simulink model "VCMGCM1962020b_v2"  (R2020b)
settings: Solver=FixedStepDiscrete  StartTime=0.0  StopTime=10.0  FixedStep=0.005  RelTol=1e-3  EnableMultiTasking=on
PreLoadFcn:
  | try, model_open; catch, disp('Error occurred while executing model pre-load callback: model_open.m'); disp('Please assure that the MATLAB working directory is set to the model directory before opening.'); end
InitFcn:
  | try, model_open; catch, end
undefined symbols (not defined in the file): Bridge, GCM, H, raptor_get_param_eval, raptor_get_safe_string, raptor_xcp_function
libraries: Blocks_lib x1165, Raptor_lib x665, simulink x62, VCM_lib x5
(part 15 of 23)

== system VCMGCM1962020b_v2/Fgnd/Actuators/CAN/CCS Interface/CCSEV_DC_ChargeInfo1/MsgTx ==
  Data : Inport
  Cmd : Inport  Port=2
  Enable : EnablePort
  Bus Selector : BusSelector  OutputSignals=VirtualSensors.Batt.BattSOC [%]
  Bus Selector1 : BusSelector  OutputSignals=EVTargetVoltage [V],EVTargetCurrent [A]
  CANTxField : Blocks_lib/CANTxField  custom=on  custom_nam=[nam '---']  custom_units='---'
  CANTxField1 : Blocks_lib/CANTxField  custom=on  custom_nam=[nam '---']  custom_units='---'
  CANTxField2 : Blocks_lib/CANTxField  custom=on  custom_nam=[nam '---']  custom_units='---'
  Header : Blocks_lib/Header  width=Landscape  addtext=''
  NO_ERROR : Constant  Value=uint8(0)
  RemainingTime : Subsystem
      settings: OpenFcn=open_system(gcb,'force')
  raptor_can_txmsg : Raptor_lib/CAN/raptor_can_txmsg  canDefinition=struct('dbcFile', 'm2iev-api.dbc','message', 'EV_DC_ChargeInfo1','comment', 'EV_DC_ChargeInfo1','signals', {{'EVErrorCode','EVRESSSOC','EVTargetVoltage','EVTargetCurrent','RemainingTimeToFullSoC','RemainingTimeToBulkSoC'}},'enabled', [ 1 1 1 1 1 1;],'canBus', 'bus','messageID', [ 256;],'idMask', [ 536870911;],'payloadMask', [],'payloadValue', [],'period', [ 50;],'mailbox', '''''','queueSize', [ 1;],'label', [ 1;],'ver', [ 2;],'showID', [ 0;],'showRaw', [ 0;],'fill', [ 0;],'editID', [ 0;],'signalOrder', [ 3;])  canBus=bus  queueSize=1  payloadMask=[]  payloadValue=[]  period=50  showID=0  label=1  idMask=hex2dec('1FFFFFFF')  fill=0  id=256  showRaw=0  signalOrder=3  signalInfo={{struct('Name', 'EVErrorCode','Startbit', [ 0;],'SignalSize', [ 4;],'ByteOrder', 'LittleEndian','ValueType', 'UNSIGNED','Class', 'uint8','Signed', [ 0;],'Factor', [ 1;],'Offset', [ 0;],'Min', [ 0;],'Max', [ 11;],'Units', 'Enum','Comment', 'Internal EV error code reported to EVSE','StartBit', [ 4;]),struct('Name', 'EVRESSSOC','Startbit', [ 0;],'SignalSize', [ 8;],'ByteOrder', 'LittleEndian','ValueType', 'UNSIGNED','Class', 'uint8','Signed', [ 0;],'Factor', [ 0.5;],'Offset', [ 0;],'Min', [ 0;],'Max', [ 127.5;],'Units', '%','Comment', 'Current state of charge','StartBit', [ 8;]),struct('Name', 'EVTargetVoltage','Startbit', [ 0;],'SignalSize', [ 16;],'ByteOrder', 'LittleEndian','ValueType', 'UNSIGNED','Class', 'uint16','Signed', [ 0;],'Factor', [ 0.05;],'Offset', [ 0;],'Min', [ 0;],'Max', [ 3276.75;],'Units', 'V','Comment', 'Voltage to be supplied by EVSE','StartBit', [ 16;]),struct('Name', 'EVTargetCurrent','Startbit', [ 0;],'SignalSize', [ 16;],'ByteOrder', 'LittleEndian','ValueType', 'SIGNED','Class', 'int16','Signed', [ 1;],'Factor', [ 0.05;],'Offset', [ 0;],'Min', [ -1638.4;],'Max', [ 1638.35;],'Units', 'A','Comment', 'Current to be supplied by EVSE','StartBit', [ 32;]),struct('Name', 'RemainingTimeToFullSoC','Startbit', [ 0;],'SignalSize', [ 8;],'ByteOrder', 'LittleEndian','ValueType', 'UNSIGNED','Class', 'uint8','Signed', [ 0;],'Factor', [ 0.5;],'Offset', [ 0;],'Min', [ 0;],'Max', [ 127.5;],'Units', 'minutes','Comment', 'Time left until charging complete','StartBit', [ 48;]),struct('Name', 'RemainingTimeToBulkSoC','Startbit', [ 0;],'SignalSize', [ 8;],'ByteOrder', 'LittleEndian','ValueType', 'UNSIGNED','Class', 'uint8','Signed', [ 0;],'Factor', [ 0.5;],'Offset', [ 0;],'Min', [ 0;],'Max', [ 127.5;],'Units', 'minutes','Comment', 'Time left until bulk charging complete','StartBit', [ 56;])}}
      settings: SourceProductName=Raptor
  wires:
  Data/1 -> Bus Selector/1, RemainingTime/1(Data)
  Bus Selector1/2 -> CANTxField2/1  "<EVTargetCurrent [A]>"
  Bus Selector1/1 -> CANTxField1/1  "<EVTargetVoltage [V]>"
  Cmd/1 -> Bus Selector1/1
  NO_ERROR/1 -> raptor_can_txmsg/1  "EVErrorCode"
  CANTxField/1 -> raptor_can_txmsg/2  "EVRESSSOC"
  CANTxField1/1 -> raptor_can_txmsg/3  "EVTargetVoltage"
  CANTxField2/1 -> raptor_can_txmsg/4  "EVTargetCurrent"
  RemainingTime/1(Full) -> raptor_can_txmsg/5  "RemainingTimeToFullSoC"
  RemainingTime/2(Bulk) -> raptor_can_txmsg/6  "RemainingTimeToBulkSoC"
  Bus Selector/1 -> CANTxField/1  "<BattSOC [%]>"

== system VCMGCM1962020b_v2/Fgnd/Actuators/CAN/CCS Interface/Commands/Charge Port DC Voltage Diag ==
  DiagEnbl : Inport
  Data : Inport  Port=2
  Bus Selector : BusSelector  OutputSignals=VirtualSensors.Chgr.ChgPortDCVoltVld [Bool]
  EvalDiag : Subsystem
  Header : Blocks_lib/Header  width=Portrait  addtext=''
  Logical Operator : Logic  AllPortsSameDT=off  OutDataTypeStr=boolean
  wires:
  Data/1 -> EvalDiag/1(Data), Bus Selector/1
  Logical Operator/1 -> EvalDiag/Enable
  Bus Selector/1 -> Logical Operator/2  "<ChgPortDCVoltVld [Bool]>"
  DiagEnbl/1 -> Logical Operator/1

== system VCMGCM1962020b_v2/Fgnd/Actuators/CAN/CCS Interface/Commands/Charge Port DC Voltage//Current ==
  Data : Inport
  Abs : Abs
  Abs1 : Abs
  Add : Sum  Inputs=+-
  Bus Selector : BusSelector  OutputSignals=VirtualSensors.Chgr.ChgPortDCVolt [V],VirtualSensors.PDU.HVBusVolt [V]
  Bus Selector1 : BusSelector  OutputSignals=VirtualSensors.Chgr.ChgPortDCVolt [V]
  Bus Selector2 : BusSelector  OutputSignals=VirtualSensors.Chgr.OffBoard.OffBoardChgrDCCur [A]
  CntrSat : Blocks_lib/CntrSat  init=0  inc=1  typ=uint16  relop=>=  th_nam='ChgPortDCVoltMatchTimeThr'  th_gain=samptime  th_units='sec'  th_help='Charge port DC voltage match (relative to HV bus voltage) time threshold'  th_group=['Actuators | CAN | ' nam]
  CntrSat1 : Blocks_lib/CntrSat  init=0  inc=1  typ=uint16  relop=>=  th_nam='ChgPortDCVoltZeroTimeThr'  th_gain=samptime  th_units='sec'  th_help='Charge port DC voltage zero time threshold'  th_group=['Actuators | CAN | ' nam]
  CntrSat2 : Blocks_lib/CntrSat  init=0  inc=1  typ=uint16  relop=>=  th_nam='ChgPortDCCurZeroTimeThr'  th_gain=samptime  th_units='sec'  th_help='Charge port DC current zero time threshold'  th_group=['Actuators | CAN | ' nam]
  Header : Blocks_lib/Header  width=Portrait  addtext=''
  Logical Operator1 : Logic  Operator=NOT  Inputs=1  OutDataTypeStr=boolean
  Logical Operator2 : Logic  Operator=NOT  Inputs=1  OutDataTypeStr=boolean
  Logical Operator3 : Logic  Operator=NOT  Inputs=1  OutDataTypeStr=boolean
  Relational Operator : RelationalOperator  Operator=<=  OutDataTypeStr=boolean  RndMeth=Nearest
  Relational Operator1 : RelationalOperator  Operator=<=  OutDataTypeStr=boolean  RndMeth=Nearest
  Relational Operator2 : RelationalOperator  Operator=<=  OutDataTypeStr=boolean  RndMeth=Nearest
  raptor_adjustment1 : Raptor_lib/Data Storage/raptor_adjustment  paramName='ChgPortDCVoltZeroThr'  nameSource=Parameter  initValue=0  dataType=double  storage=Calibration  calDispType=Number  calEnum={'Disabled', 'Enabled'}  calGain=1  calOffset=0  calMax=inf  calMin=-inf  calFormat=''  calUnit='V'  calHelp='Charge port DC voltage zero threshold'  calAccess=1  calFunction=['Actuators | CAN | ' nam]  calDispHeaders=off  calColHeaders={'Col1' 'Col2' 'Col3'}  calRowHeaders={'Row1' 'Row2' 'Row3'}
      settings: SourceProductName=Raptor
  raptor_adjustment2 : Raptor_lib/Data Storage/raptor_adjustment  paramName='ChgPortDCCurZeroThr'  nameSource=Parameter  initValue=0  dataType=double  storage=Calibration  calDispType=Number  calEnum={'Disabled', 'Enabled'}  calGain=1  calOffset=0  calMax=inf  calMin=-inf  calFormat=''  calUnit='A'  calHelp='Charge port DC current zero threshold'  calAccess=1  calFunction=['Actuators | CAN | ' nam]  calDispHeaders=off  calColHeaders={'Col1' 'Col2' 'Col3'}  calRowHeaders={'Row1' 'Row2' 'Row3'}
      settings: SourceProductName=Raptor
  raptor_adjustment5 : Raptor_lib/Data Storage/raptor_adjustment  paramName='ChgPortDCVoltMatchThr'  nameSource=Parameter  initValue=0  dataType=double  storage=Calibration  calDispType=Number  calEnum={'Disabled', 'Enabled'}  calGain=1  calOffset=0  calMax=inf  calMin=-inf  calFormat=''  calUnit='V'  calHelp='Charge port DC voltage match (relative to HV bus voltage) threshold'  calAccess=1  calFunction=['Actuators | CAN | ' nam]  calDispHeaders=off  calColHeaders={'Col1' 'Col2' 'Col3'}  calRowHeaders={'Row1' 'Row2' 'Row3'}
      settings: SourceProductName=Raptor
  VoltMatch : Outport  VectorParamsAs1DForOutWhenUnconnected=off
  VoltZero : Outport  Port=2  VectorParamsAs1DForOutWhenUnconnected=off
  CurZero : Outport  Port=3  VectorParamsAs1DForOutWhenUnconnected=off
  wires:
  Relational Operator/1 -> Logical Operator3/1, CntrSat/1
  CntrSat/1 -> VoltMatch/1
  Logical Operator3/1 -> CntrSat/2
  Abs1/1 -> Relational Operator2/1
  Bus Selector2/1 -> Abs1/1  "<OffBoardChgrDCCur [A]>"
  raptor_adjustment2/1 -> Relational Operator2/2
  Data/1 -> Bus Selector/1, Bus Selector1/1, Bus Selector2/1
  Bus Selector1/1 -> Relational Operator1/1  "<ChgPortDCVolt [V]>"
  Abs/1 -> Relational Operator/1
  Add/1 -> Abs/1
  Bus Selector/2 -> Add/2  "<HVBusVolt [V]>"
  Bus Selector/1 -> Add/1  "<ChgPortDCVolt [V]>"
  raptor_adjustment1/1 -> Relational Operator1/2
  raptor_adjustment5/1 -> Relational Operator/2
  Logical Operator1/1 -> CntrSat1/2
  CntrSat1/1 -> VoltZero/1
  Relational Operator1/1 -> CntrSat1/1, Logical Operator1/1
  Relational Operator2/1 -> Logical Operator2/1, CntrSat2/1
  CntrSat2/1 -> CurZero/1
  Logical Operator2/1 -> CntrSat2/2

== system VCMGCM1962020b_v2/Fgnd/Actuators/CAN/CCS Interface/Commands/DC Charge Contactors ==
  Data : Inport
  Bus Selector : BusSelector  OutputSignals=VirtualSensors.PDU.DCDCCntrClosed [Bool],VirtualSensors.PDU.DCChgNegCntrClosed [Bool]
  Header : Blocks_lib/Header  width=Portrait  addtext=''
  Logical Operator : Logic  AllPortsSameDT=off  OutDataTypeStr=boolean
  Logical Operator1 : Logic  AllPortsSameDT=off  OutDataTypeStr=boolean
  Logical Operator2 : Logic  Operator=NOT  Inputs=1  AllPortsSameDT=off  OutDataTypeStr=boolean
  Logical Operator3 : Logic  Operator=NOT  Inputs=1  AllPortsSameDT=off  OutDataTypeStr=boolean
  Closed : Outport  VectorParamsAs1DForOutWhenUnconnected=off
  Open : Outport  Port=2  VectorParamsAs1DForOutWhenUnconnected=off
  wires:
  Logical Operator3/1 -> Logical Operator1/2
  Logical Operator2/1 -> Logical Operator1/1
  Bus Selector/2 -> Logical Operator/2, Logical Operator3/1  "<DCChgNegCntrClosed [Bool]>"
  Bus Selector/1 -> Logical Operator/1, Logical Operator2/1  "<DCDCCntrClosed [Bool]>"
  Data/1 -> Bus Selector/1
  Logical Operator/1 -> Closed/1
  Logical Operator1/1 -> Open/1

== system VCMGCM1962020b_v2/Fgnd/Actuators/CAN/CCS Interface/MsgName/MsgTx ==
  Cmd : Inport
  Enable : EnablePort
  Bus Selector : BusSelector  OutputSignals=Command [enum],DC_ContactorsState [Bool]
  CANTxField : Blocks_lib/CANTxField  custom=on  custom_nam=[nam '---']  custom_units='---'
  CANTxField1 : Blocks_lib/CANTxField  custom=on  custom_nam=[nam '---']  custom_units='---'
  Header : Blocks_lib/Header  width=Landscape  addtext=''
  OPEN : Constant  Value=uint8(0)
  Vendor-specific error code : Constant  Value=uint8(0)
  Vendor-specific error info : Constant  Value=uint8(0)
  Vendor-specific state : Constant  Value=uint8(0)
  raptor_can_txmsg : Raptor_lib/CAN/raptor_can_txmsg  canDefinition=struct('dbcFile', 'm2iev-api.dbc','message', 'BCC_Command','comment', 'BCC_Command','signals', {{'CurrentState','Command','AC_ContactorsState','DC_ContactorsState','ErrorCode','ErrorInfo'}},'enabled', [ 1 1 1 1 1 1;],'canBus', 'bus','messageID', [ 128;],'idMask', [ 536870911;],'payloadMask', [],'payloadValue', [],'period', [ 50;],'mailbox', '''''','queueSize', [ 1;],'label', [ 1;],'ver', [ 2;],'showID', [ 0;],'showRaw', [ 0;],'fill', [ 0;],'editID', [ 0;],'signalOrder', [ 3;])  canBus=bus  queueSize=1  payloadMask=[]  payloadValue=[]  period=50  showID=0  label=1  idMask=hex2dec('1FFFFFFF')  fill=0  id=128  showRaw=0  signalOrder=3  signalInfo={{struct('Name', 'CurrentState','Startbit', [ 0;],'SignalSize', [ 8;],'ByteOrder', 'LittleEndian','ValueType', 'UNSIGNED','Class', 'uint8','Signed', [ 0;],'Factor', [ 1;],'Offset', [ 0;],'Min', [ 0;],'Max', [ 255;],'Units', 'Enum','Comment', 'Current state of BCC (vendor specific). Is not analyzed but logged to get overall picture','StartBit', [ 0;]),struct('Name', 'Command','Startbit', [ 0;],'SignalSize', [ 4;],'ByteOrder', 'LittleEndian','ValueType', 'UNSIGNED','Class', 'uint8','Signed', [ 0;],'Factor', [ 1;],'Offset', [ 0;],'Min', [ 0;],'Max', [ 8;],'Units', 'Enum','Comment', 'Command from BCC to M2IEV (used to start, stop charging, putting the module into low power modes and etc.)','StartBit', [ 8;]),struct('Name', 'AC_ContactorsState','Startbit', [ 0;],'SignalSize', [ 1;],'ByteOrder', 'LittleEndian','ValueType', 'UNSIGNED','Class', 'uint8','Signed', [ 0;],'Factor', [ 1;],'Offset', [ 0;],'Min', [ 0;],'Max', [ 1;],'Units', 'Boolean','Comment', 'Current state of AC contactors','StartBit', [ 13;]),struct('Name', 'DC_ContactorsState','Startbit', [ 0;],'SignalSize', [ 1;],'ByteOrder', 'LittleEndian','ValueType', 'UNSIGNED','Class', 'uint8','Signed', [ 0;],'Factor', [ 1;],'Offset', [ 0;],'Min', [ 0;],'Max', [ 1;],'Units', 'Boolean','Comment', 'Current state of DC contactors','StartBit', [ 14;]),struct('Name', 'ErrorCode','Startbit', [ 0;],'SignalSize', [ 8;],'ByteOrder', 'LittleEndian','ValueType', 'UNSIGNED','Class', 'uint8','Signed', [ 0;],'Factor', [ 1;],'Offset', [ 0;],'Min', [ 0;],'Max', [ 255;],'Units', 'Enum','Comment', 'Internal BCC error code (vendor specific)','StartBit', [ 17;]),struct('Name', 'ErrorInfo','Startbit', [ 0;],'SignalSize', [ 8;],'ByteOrder', 'LittleEndian','ValueType', 'UNSIGNED','Class', 'uint8','Signed', [ 0;],'Factor', [ 1;],'Offset', [ 0;],'Min', [ 0;],'Max', [ 255;],'Units', 'Enum','Comment', 'Supplementary error information','StartBit', [ 25;])}}
      settings: SourceProductName=Raptor
  wires:
  Bus Selector/2 -> CANTxField1/1  "<DC_ContactorsState [Bool]>"
  Bus Selector/1 -> CANTxField/1  "<Command [enum]>"
  Cmd/1 -> Bus Selector/1
  Vendor-specific error info/1 -> raptor_can_txmsg/6  "ErrorInfo"
  Vendor-specific error code/1 -> raptor_can_txmsg/5  "ErrorCode"
  CANTxField1/1 -> raptor_can_txmsg/4  "DC_ContactorsState"
  OPEN/1 -> raptor_can_txmsg/3  "AC_ContactorsState"
  CANTxField/1 -> raptor_can_txmsg/2  "Command"
  Vendor-specific state/1 -> raptor_can_txmsg/1  "CurrentState"

== system VCMGCM1962020b_v2/Fgnd/Actuators/CAN/CCS Interface/MsgName/SleepMsgTx ==
  Trigger : TriggerPort  TriggerType=falling  VariantControl=Variant  PortDimensions=1
  Header : Blocks_lib/Header  width=Landscape  addtext=''
  OPEN : Constant  Value=uint8(0)
  "OPEN " : Constant  Value=uint8(0)
  Sleep : Constant  Value=uint8(1)
  Vendor-specific error code : Constant  Value=uint8(0)
  Vendor-specific error info : Constant  Value=uint8(0)
  Vendor-specific state : Constant  Value=uint8(0)
  raptor_can_txmsg : Raptor_lib/CAN/raptor_can_txmsg  canDefinition=struct('dbcFile', 'm2iev-api.dbc','message', 'BCC_Command','comment', 'BCC_Command','signals', {{'CurrentState','Command','AC_ContactorsState','DC_ContactorsState','ErrorCode','ErrorInfo'}},'enabled', [ 1 1 1 1 1 1;],'canBus', 'bus','messageID', [ 128;],'idMask', [ 536870911;],'payloadMask', [],'payloadValue', [],'period', [ 50;],'mailbox', '''''','queueSize', [ 1;],'label', [ 1;],'ver', [ 2;],'showID', [ 0;],'showRaw', [ 0;],'fill', [ 0;],'editID', [ 0;],'signalOrder', [ 3;])  canBus=bus  queueSize=1  payloadMask=[]  payloadValue=[]  period=50  showID=0  label=1  idMask=hex2dec('1FFFFFFF')  fill=0  id=128  showRaw=0  signalOrder=3  signalInfo={{struct('Name', 'CurrentState','Startbit', [ 0;],'SignalSize', [ 8;],'ByteOrder', 'LittleEndian','ValueType', 'UNSIGNED','Class', 'uint8','Signed', [ 0;],'Factor', [ 1;],'Offset', [ 0;],'Min', [ 0;],'Max', [ 255;],'Units', 'Enum','Comment', 'Current state of BCC (vendor specific). Is not analyzed but logged to get overall picture','StartBit', [ 0;]),struct('Name', 'Command','Startbit', [ 0;],'SignalSize', [ 4;],'ByteOrder', 'LittleEndian','ValueType', 'UNSIGNED','Class', 'uint8','Signed', [ 0;],'Factor', [ 1;],'Offset', [ 0;],'Min', [ 0;],'Max', [ 8;],'Units', 'Enum','Comment', 'Command from BCC to M2IEV (used to start, stop charging, putting the module into low power modes and etc.)','StartBit', [ 8;]),struct('Name', 'AC_ContactorsState','Startbit', [ 0;],'SignalSize', [ 1;],'ByteOrder', 'LittleEndian','ValueType', 'UNSIGNED','Class', 'uint8','Signed', [ 0;],'Factor', [ 1;],'Offset', [ 0;],'Min', [ 0;],'Max', [ 1;],'Units', 'Boolean','Comment', 'Current state of AC contactors','StartBit', [ 13;]),struct('Name', 'DC_ContactorsState','Startbit', [ 0;],'SignalSize', [ 1;],'ByteOrder', 'LittleEndian','ValueType', 'UNSIGNED','Class', 'uint8','Signed', [ 0;],'Factor', [ 1;],'Offset', [ 0;],'Min', [ 0;],'Max', [ 1;],'Units', 'Boolean','Comment', 'Current state of DC contactors','StartBit', [ 14;]),struct('Name', 'ErrorCode','Startbit', [ 0;],'SignalSize', [ 8;],'ByteOrder', 'LittleEndian','ValueType', 'UNSIGNED','Class', 'uint8','Signed', [ 0;],'Factor', [ 1;],'Offset', [ 0;],'Min', [ 0;],'Max', [ 255;],'Units', 'Enum','Comment', 'Internal BCC error code (vendor specific)','StartBit', [ 17;]),struct('Name', 'ErrorInfo','Startbit', [ 0;],'SignalSize', [ 8;],'ByteOrder', 'LittleEndian','ValueType', 'UNSIGNED','Class', 'uint8','Signed', [ 0;],'Factor', [ 1;],'Offset', [ 0;],'Min', [ 0;],'Max', [ 255;],'Units', 'Enum','Comment', 'Supplementary error information','StartBit', [ 25;])}}
      settings: SourceProductName=Raptor
  wires:
  Vendor-specific state/1 -> raptor_can_txmsg/1  "CurrentState"
  Sleep/1 -> raptor_can_txmsg/2  "Command"
  OPEN/1 -> raptor_can_txmsg/3  "AC_ContactorsState"
  "OPEN "/1 -> raptor_can_txmsg/4  "DC_ContactorsState"
  Vendor-specific error code/1 -> raptor_can_txmsg/5  "ErrorCode"
  Vendor-specific error info/1 -> raptor_can_txmsg/6  "ErrorInfo"

== system VCMGCM1962020b_v2/Fgnd/Actuators/CAN/Charger/ChgrBMSA/MsgTx ==
  Data : Inport
  Enable : EnablePort
  Bus Selector : BusSelector  OutputSignals=Control.Batt.MaxVoltAllow,Control.Chgr.OnBoardChgrDCCurLim [A],Control.Chgr.OnBoardChgrEnblReq [Bool]
  CANTxField{,1..3} (4 alike) : Blocks_lib/CANTxField  custom=on  custom_nam=[nam '---']  custom_units='---'
  Constant : Constant  Value=0
  Header : Blocks_lib/Header  width=Landscape  addtext=''
  NOT : Logic  Operator=NOT  AllPortsSameDT=off  OutDataTypeStr=boolean
  raptor_can_txmsg : Raptor_lib/CAN/raptor_can_txmsg  canDefinition=struct('dbcFile', 'Dilong Digital Charger_dbc file.dbc','message', 'BMSA','comment', 'Battery management system','signals', {{'Max_allow_chrg_volt','Max_allow_chrg_curr','Chrg_cmmd','Batt_mode'}},'enabled', [ 1 1 1 1;],'scaled', [ 1 1 1 1;],'canBus', 'bus','messageID', [ 403105268;],'idMask', [ 536870911;],'payloadMask', [],'payloadValue', [],'period', [ 100;],'mailbox', '''''','queueSize', [ 1;],'label', [ 1;],'ver', [ 2;],'showID', [ 0;],'showRaw', [ 0;],'showRawMsg', [ 0;],'fill', [ 0;],'editID', [ 0;],'signalOrder', [ 3;],'signalAscDes', [ 1;])  canBus=bus  queueSize=1  payloadMask=[]  payloadValue=[]  period=100  showID=0  label=1  idMask=hex2dec('1FFFFFFF')  fill=0  id=403105268  showRaw=0  signalOrder=3  signalInfo={{struct('Name', 'Max_allow_chrg_volt','Startbit', [ 0;],'SignalSize', [ 16;],'ByteOrder', 'BigEndian','ValueType', 'UNSIGNED','Class', 'uint16','Signed', [ 0;],'Factor', [ 0.1;],'Offset', [ 0;],'Min', [ 0;],'Max', [ 1320;],'Units', 'V','Comment', '','StartBit', [ 8;]),struct('Name', 'Max_allow_chrg_curr','Startbit', [ 0;],'SignalSize', [ 16;],'ByteOrder', 'BigEndian','ValueType', 'UNSIGNED','Class', 'uint16','Signed', [ 0;],'Factor', [ 0.1;],'Offset', [ 0;],'Min', [ 0;],'Max', [ 350;],'Units', 'A','Comment', '','StartBit', [ 24;]),struct('Name', 'Chrg_cmmd','Startbit', [ 0;],'SignalSize', [ 8;],'ByteOrder', 'BigEndian','ValueType', 'UNSIGNED','Class', 'uint8','Signed', [ 0;],'Factor', [ 1;],'Offset', [ 0;],'Min', [ 0;],'Max', [ 2;],'Units', 'enum','Comment', '','StartBit', [ 32;]),struct('Name', 'Batt_mode','Startbit', [ 0;],'SignalSize', [ 8;],'ByteOrder', 'BigEndian','ValueType', 'UNSIGNED','Class', 'uint8','Signed', [ 0;],'Factor', [ 1;],'Offset', [ 0;],'Min', [ 0;],'Max', [ 1;],'Units', 'enum','Comment', '','StartBit', [ 40;])}}
      settings: SourceProductName=Raptor
  wires:
  CANTxField/1 -> raptor_can_txmsg/1  "Max_allow_chrg_volt"
  CANTxField1/1 -> raptor_can_txmsg/2  "Max_allow_chrg_curr"
  CANTxField3/1 -> raptor_can_txmsg/4  "Batt_mode"
  CANTxField2/1 -> raptor_can_txmsg/3  "Chrg_cmmd"
  Data/1 -> Bus Selector/1
  Bus Selector/3 -> NOT/1  "<OnBoardChgrEnblReq [Bool]>"
  NOT/1 -> CANTxField2/1
  Bus Selector/2 -> CANTxField1/1  "<OnBoardChgrDCCurLim [A]>"
  Bus Selector/1 -> CANTxField/1  "<MaxVoltAllow>"
  Constant/1 -> CANTxField3/1

== system VCMGCM1962020b_v2/Fgnd/Actuators/CAN/Charger/Config Msgs/Config Sequence ==
  note: Note: per EDN, the 0x616 message is only transmitted once when power is first applied to the charger.
      | So, unplug/plug the charger connector to get the 0x616 message.
      | Then, immediately prompt the configuration sequence by setting ChgrConfigPrompt = 1.
  Enable : EnablePort
  0x616 : Subsystem
  0x617_00 : Subsystem
  0x617_A5 : Subsystem
  Config Sequence : Stateflow chart  TreatAsAtomicUnit=on
  Header : Blocks_lib/Header  width=Portrait  addtext=''
  raptor_adjustment : Raptor_lib/Data Storage/raptor_adjustment  paramName='ChgrConfigMxTime'  nameSource=Parameter  initValue=0  dataType=uint16  storage=Calibration  calDispType=Number  calEnum={}  calGain=samptime  calOffset=0  calMax=inf  calMin=-inf  calFormat='0.3'  calUnit='sec'  calHelp='Charger configuration maximum time'  calAccess=1  calFunction='Actuators | CAN | ChgrConfig'  calDispHeaders=off  calColHeaders={'Col1' 'Col2' 'Col3'}  calRowHeaders={'Row1' 'Row2' 'Row3'}
      settings: SourceProductName=Raptor
  raptor_adjustment1 : Raptor_lib/Data Storage/raptor_adjustment  paramName='ChgrConfigTxRate'  nameSource=Parameter  initValue=0  dataType=uint16  storage=Calibration  calDispType=Number  calEnum={}  calGain=samptime  calOffset=0  calMax=inf  calMin=-inf  calFormat='0.3'  calUnit='sec'  calHelp='Charger configuration message transmit rate'  calAccess=1  calFunction='Actuators | CAN | ChgrConfig'  calDispHeaders=off  calColHeaders={'Col1' 'Col2' 'Col3'}  calRowHeaders={'Row1' 'Row2' 'Row3'}
      settings: SourceProductName=Raptor
  raptor_can_trigger : Raptor_lib/CAN/raptor_can_trigger  mailbox='Chgr616Msg'  inherited=1  alwaysEnabled=0  triggerPriority=0
      settings: SourceProductName=Raptor
  raptor_data_def : Raptor_lib/Data Storage/raptor_data_def  dataName='ChgrConfigPrompt'  initValue=0  dataType=boolean  storage=Volatile (RAM)  calVisible=on  calType=Adjustment  calDispType=Number  calEnum={}  calGain=1  calOffset=0  calMin=-inf  calMax=inf  calFormat=''  calUnit='Bool'  calHelp='Charger configuration prompt'  calAccess=1  calFunction='Actuators | CAN | ChgrConfig'  calDispHeaders=off  calColHeaders={'Col1' 'Col2' 'Col3'}  calRowHeaders={'Row1' 'Row2' 'Row3'}
      settings: SourceProductName=Raptor
  raptor_data_read : Raptor_lib/Data Storage/raptor_data_read  dataName='ChgrConfigComplete'  dataShape=Scalar  idxSource=Input  idxRow=1  idxCol=1
      settings: SourceProductName=Raptor
  raptor_data_read1 : Raptor_lib/Data Storage/raptor_data_read  dataName='ChgrConfigPrompt'  dataShape=Scalar  idxSource=Input  idxRow=1  idxCol=1
      settings: SourceProductName=Raptor
  wires:
  Config Sequence/1(Tx617_A5()) -> 0x617_A5/Trigger
  Config Sequence/2(Tx617_00()) -> 0x617_00/Trigger
  raptor_adjustment/1 -> Config Sequence/3(MxTime)
  raptor_adjustment1/1 -> Config Sequence/4(TxRate)
  raptor_data_read1/1 -> Config Sequence/1(ConfigPrompt)
  raptor_data_read/1 -> Config Sequence/2(ConfigComplete)
  raptor_can_trigger/1 -> 0x616/Trigger

== system VCMGCM1962020b_v2/Fgnd/Actuators/CAN/DC//DC Converter/MsgName/MsgTx ==
  Data : Inport
  Enable : EnablePort
  Bus Selector2 : BusSelector  OutputSignals=Control.DCDC.DCDCOutptCurLim [A],Control.DCDC.DCDCOutptVoltSetpt [V],Control.DCDC.DCDCEnblReq [Bool]
  CANTxField : Blocks_lib/CANTxField  custom=on  custom_nam=[nam '---']  custom_units='---'
  CANTxField1 : Blocks_lib/CANTxField  custom=on  custom_nam=[nam '---']  custom_units='---'
  CANTxField2 : Blocks_lib/CANTxField  custom=on  custom_nam=[nam '---']  custom_units='---'
  Header : Blocks_lib/Header  width=Landscape  addtext=''
  raptor_adjustment : Raptor_lib/Data Storage/raptor_adjustment  paramName=[nam 'OutputOVLimit']  nameSource=Parameter  initValue=18  dataType=double  storage=Calibration  calDispType=Number  calEnum={'Disabled', 'Enabled'}  calGain=1  calOffset=0  calMax=inf  calMin=-inf  calFormat=''  calUnit='V'  calHelp='Output over-voltage limit'  calAccess=1  calFunction=['Actuators | CAN | ' msgnam]  calDispHeaders=off  calColHeaders={'Col1' 'Col2' 'Col3'}  calRowHeaders={'Row1' 'Row2' 'Row3'}
      settings: SourceProductName=Raptor
  raptor_adjustment1 : Raptor_lib/Data Storage/raptor_adjustment  paramName=[nam 'OutputUVLimit']  nameSource=Parameter  initValue=8  dataType=double  storage=Calibration  calDispType=Number  calEnum={'Disabled', 'Enabled'}  calGain=1  calOffset=0  calMax=inf  calMin=-inf  calFormat=''  calUnit='V'  calHelp='Output under-voltage limit'  calAccess=1  calFunction=['Actuators | CAN | ' msgnam]  calDispHeaders=off  calColHeaders={'Col1' 'Col2' 'Col3'}  calRowHeaders={'Row1' 'Row2' 'Row3'}
      settings: SourceProductName=Raptor
  raptor_adjustment2 : Raptor_lib/Data Storage/raptor_adjustment  paramName=[nam 'CoolingPlateFaultLim']  nameSource=Parameter  initValue=75  dataType=double  storage=Calibration  calDispType=Number  calEnum={'Disabled', 'Enabled'}  calGain=1  calOffset=0  calMax=inf  calMin=-inf  calFormat=''  calUnit='degC'  calHelp='Cooling plate fault limit'  calAccess=1  calFunction=['Actuators | CAN | ' msgnam]  calDispHeaders=off  calColHeaders={'Col1' 'Col2' 'Col3'}  calRowHeaders={'Row1' 'Row2' 'Row3'}
      settings: SourceProductName=Raptor
  raptor_adjustment3 : Raptor_lib/Data Storage/raptor_adjustment  paramName=[nam 'CoolingPlateWarningLim']  nameSource=Parameter  initValue=60  dataType=double  storage=Calibration  calDispType=Number  calEnum={'Disabled', 'Enabled'}  calGain=1  calOffset=0  calMax=inf  calMin=-inf  calFormat=''  calUnit='degC'  calHelp='Cooling plate warning limit'  calAccess=1  calFunction=['Actuators | CAN | ' msgnam]  calDispHeaders=off  calColHeaders={'Col1' 'Col2' 'Col3'}  calRowHeaders={'Row1' 'Row2' 'Row3'}
      settings: SourceProductName=Raptor
  raptor_can_txmsg : Raptor_lib/CAN/raptor_can_txmsg  canDefinition=struct('dbcFile', 'BelPwrDCDC.dbc','message', 'OutputSetpoint:0','comment', '','signals', {{'CoolingPlateFaultLim','CoolingPlateWarningLim','Mode','OutputCurrentSetpt','OutputOVLimit','OutputUVLimit','OutputVoltageSetpt','RemoteShutdown'}},'enabled', [ 0 0 0 1 0 0 1 1;],'canBus', 'bus','messageID', [ 418362112;],'idMask', [ 536870911;],'payloadMask', [],'payloadValue', [],'period', [ 100;],'mailbox', '''''','queueSize', [ 1;],'label', [ 1;],'ver', [ 2;],'showID', [ 0;],'showRaw', [ 0;],'fill', [ 0;],'editID', [ 0;],'signalOrder', [ 1;])  canBus=bus  queueSize=1  payloadMask=[]  payloadValue=[]  period=100  showID=0  label=1  idMask=hex2dec('1FFFFFFF')  fill=0  id=418362112  showRaw=0  signalOrder=1  signalInfo={{struct('Name', 'OutputVoltageSetpt','Startbit', [ 0;],'SignalSize', [ 16;],'ByteOrder', 'LittleEndian','ValueType', 'UNSIGNED','Class', 'uint16','Signed', [ 0;],'Factor', [ 0.05;],'Offset', [ 0;],'Min', [ 0;],'Max', [ 3276.75;],'Units', 'V','Comment', '','StartBit', [ 8;]),struct('Name', 'Mode','Startbit', [ 0;],'SignalSize', [ 8;],'ByteOrder', 'LittleEndian','ValueType', 'UNSIGNED','Class', 'uint8','Signed', [ 0;],'Factor', [ 1;],'Offset', [ 0;],'Min', [ 0;],'Max', [ 3;],'Units', 'enum','Comment', '','StartBit', [ 0;]),struct('Name', 'OutputCurrentSetpt','Startbit', [ 0;],'SignalSize', [ 16;],'ByteOrder', 'LittleEndian','ValueType', 'UNSIGNED','Class', 'uint16','Signed', [ 0;],'Factor', [ 0.05;],'Offset', [ 0;],'Min', [ 0;],'Max', [ 3276.75;],'Units', 'A','Comment', '','StartBit', [ 24;]),struct('Name', 'RemoteShutdown','Startbit', [ 0;],'SignalSize', [ 8;],'ByteOrder', 'LittleEndian','ValueType', 'UNSIGNED','Class', 'uint8','Signed', [ 0;],'Factor', [ 1;],'Offset', [ 0;],'Min', [ 0;],'Max', [ 1;],'Units', 'bool','Comment', '','StartBit', [ 40;]),struct('Name', 'OutputUVLimit','Startbit', [ 0;],'SignalSize', [ 16;],'ByteOrder', 'LittleEndian','ValueType', 'UNSIGNED','Class', 'uint16','Signed', [ 0;],'Factor', [ 0.05;],'Offset', [ 0;],'Min', [ 0;],'Max', [ 3276.75;],'Units', 'V','Comment', '','StartBit', [ 8;]),struct('Name', 'OutputOVLimit','Startbit', [ 0;],'SignalSize', [ 16;],'ByteOrder', 'LittleEndian','ValueType', 'UNSIGNED','Class', 'uint16','Signed', [ 0;],'Factor', [ 0.05;],'Offset', [ 0;],'Min', [ 0;],'Max', [ 3276.75;],'Units', 'V','Comment', '','StartBit', [ 24;]),struct('Name', 'CoolingPlateFaultLim','Startbit', [ 0;],'SignalSize', [ 16;],'ByteOrder', 'LittleEndian','ValueType', 'SIGNED','Class', 'int16','Signed', [ 1;],'Factor', [ 0.1;],'Offset', [ 0;],'Min', [ -3276.8;],'Max', [ 3276.7;],'Units', 'degC','Comment', '','StartBit', [ 8;]),struct('Name', 'CoolingPlateWarningLim','Startbit', [ 0;],'SignalSize', [ 16;],'ByteOrder', 'LittleEndian','ValueType', 'SIGNED','Class', 'int16','Signed', [ 1;],'Factor', [ 0.1;],'Offset', [ 0;],'Min', [ -3276.8;],'Max', [ 3276.7;],'Units', 'degC','Comment', '','StartBit', [ 24;])}}
      settings: SourceProductName=Raptor
  raptor_can_txmsg1 : Raptor_lib/CAN/raptor_can_txmsg  canDefinition=struct('dbcFile', 'BelPwrDCDC.dbc','message', 'OutputSetpoint:1','comment', '','signals', {{'CoolingPlateFaultLim','CoolingPlateWarningLim','Mode','OutputCurrentSetpt','OutputOVLimit','OutputUVLimit','OutputVoltageSetpt','RemoteShutdown'}},'enabled', [ 0 0 0 0 1 1 0 0;],'scaled', [ 0 0 1 0 1 1 0 0;],'canBus', 'bus','messageID', [ 418362112;],'idMask', [ 536870911;],'payloadMask', [],'payloadValue', [],'period', [ 100;],'mailbox', '''''','queueSize', [ 1;],'label', [ 1;],'ver', [ 2;],'showID', [ 0;],'showRaw', [ 0;],'fill', [ 0;],'editID', [ 0;],'signalOrder', [ 1;],'signalAscDes', [ 1;])  canBus=bus  queueSize=1  payloadMask=[]  payloadValue=[]  period=100  showID=0  label=1  idMask=hex2dec('1FFFFFFF')  fill=0  id=418362112  showRaw=0  signalOrder=1  signalInfo={{struct('Name', 'OutputVoltageSetpt','Startbit', [ 0;],'SignalSize', [ 16;],'ByteOrder', 'LittleEndian','ValueType', 'UNSIGNED','Class', 'uint16','Signed', [ 0;],'Factor', [ 1;],'Offset', [ 0;],'Min', [ 0;],'Max', [ 65535;],'Units', '','Comment', '','StartBit', [ 8;]),struct('Name', 'Mode','Startbit', [ 0;],'SignalSize', [ 8;],'ByteOrder', 'LittleEndian','ValueType', 'UNSIGNED','Class', 'uint8','Signed', [ 0;],'Factor', [ 1;],'Offset', [ 0;],'Min', [ 0;],'Max', [ 255;],'Units', '','Comment', '','StartBit', [ 0;]),struct('Name', 'OutputCurrentSetpt','Startbit', [ 0;],'SignalSize', [ 16;],'ByteOrder', 'LittleEndian','ValueType', 'UNSIGNED','Class', 'uint16','Signed', [ 0;],'Factor', [ 0.05;],'Offset', [ 0;],'Min', [ 0;],'Max', [ 3276.75;],'Units', 'A','Comment', '','StartBit', [ 24;]),struct('Name', 'RemoteShutdown','Startbit', [ 0;],'SignalSize', [ 8;],'ByteOrder', 'LittleEndian','ValueType', 'UNSIGNED','Class', 'uint8','Signed', [ 0;],'Factor', [ 1;],'Offset', [ 0;],'Min', [ 0;],'Max', [ 255;],'Units', '','Comment', '','StartBit', [ 40;]),struct('Name', 'OutputUVLimit','Startbit', [ 0;],'SignalSize', [ 16;],'ByteOrder', 'LittleEndian','ValueType', 'UNSIGNED','Class', 'uint16','Signed', [ 0;],'Factor', [ 0.05;],'Offset', [ 0;],'Min', [ 0;],'Max', [ 3276.75;],'Units', 'V','Comment', '','StartBit', [ 8;]),struct('Name', 'OutputOVLimit','Startbit', [ 0;],'SignalSize', [ 16;],'ByteOrder', 'LittleEndian','ValueType', 'UNSIGNED','Class', 'uint16','Signed', [ 0;],'Factor', [ 0.05;],'Offset', [ 0;],'Min', [ 0;],'Max', [ 3276.75;],'Units', 'V','Comment', '','StartBit', [ 24;]),struct('Name', 'CoolingPlateFaultLim','Startbit', [ 0;],'SignalSize', [ 16;],'ByteOrder', 'LittleEndian','ValueType', 'SIGNED','Class', 'int16','Signed', [ 1;],'Factor', [ 1;],'Offset', [ 0;],'Min', [ -32768;],'Max', [ 32767;],'Units', '','Comment', '','StartBit', [ 8;]),struct('Name', 'CoolingPlateWarningLim','Startbit', [ 0;],'SignalSize', [ 16;],'ByteOrder', 'LittleEndian','ValueType', 'SIGNED','Class', 'int16','Signed', [ 1;],'Factor', [ 1;],'Offset', [ 0;],'Min', [ -32768;],'Max', [ 32767;],'Units', '','Comment', '','StartBit', [ 24;])}}
      settings: SourceProductName=Raptor
  raptor_can_txmsg2 : Raptor_lib/CAN/raptor_can_txmsg  canDefinition=struct('dbcFile', 'BelPwrDCDC.dbc','message', 'OutputSetpoint:2','comment', '','signals', {{'CoolingPlateFaultLim','CoolingPlateWarningLim','Mode','OutputCurrentSetpt','OutputOVLimit','OutputUVLimit','OutputVoltageSetpt','RemoteShutdown'}},'enabled', [ 1 1 0 0 0 0 0 0;],'canBus', 'bus','messageID', [ 418362112;],'idMask', [ 536870911;],'payloadMask', [],'payloadValue', [],'period', [ 100;],'mailbox', '''''','queueSize', [ 1;],'label', [ 1;],'ver', [ 2;],'showID', [ 0;],'showRaw', [ 0;],'fill', [ 0;],'editID', [ 0;],'signalOrder', [ 1;])  canBus=bus  queueSize=1  payloadMask=[]  payloadValue=[]  period=100  showID=0  label=1  idMask=hex2dec('1FFFFFFF')  fill=0  id=418362112  showRaw=0  signalOrder=1  signalInfo={{struct('Name', 'OutputVoltageSetpt','Startbit', [ 0;],'SignalSize', [ 16;],'ByteOrder', 'LittleEndian','ValueType', 'UNSIGNED','Class', 'uint16','Signed', [ 0;],'Factor', [ 0.05;],'Offset', [ 0;],'Min', [ 0;],'Max', [ 3276.75;],'Units', 'V','Comment', '','StartBit', [ 8;]),struct('Name', 'Mode','Startbit', [ 0;],'SignalSize', [ 8;],'ByteOrder', 'LittleEndian','ValueType', 'UNSIGNED','Class', 'uint8','Signed', [ 0;],'Factor', [ 1;],'Offset', [ 0;],'Min', [ 0;],'Max', [ 3;],'Units', 'enum','Comment', '','StartBit', [ 0;]),struct('Name', 'OutputCurrentSetpt','Startbit', [ 0;],'SignalSize', [ 16;],'ByteOrder', 'LittleEndian','ValueType', 'UNSIGNED','Class', 'uint16','Signed', [ 0;],'Factor', [ 0.05;],'Offset', [ 0;],'Min', [ 0;],'Max', [ 3276.75;],'Units', 'A','Comment', '','StartBit', [ 24;]),struct('Name', 'RemoteShutdown','Startbit', [ 0;],'SignalSize', [ 8;],'ByteOrder', 'LittleEndian','ValueType', 'UNSIGNED','Class', 'uint8','Signed', [ 0;],'Factor', [ 1;],'Offset', [ 0;],'Min', [ 0;],'Max', [ 1;],'Units', 'bool','Comment', '','StartBit', [ 40;]),struct('Name', 'OutputUVLimit','Startbit', [ 0;],'SignalSize', [ 16;],'ByteOrder', 'LittleEndian','ValueType', 'UNSIGNED','Class', 'uint16','Signed', [ 0;],'Factor', [ 0.05;],'Offset', [ 0;],'Min', [ 0;],'Max', [ 3276.75;],'Units', 'V','Comment', '','StartBit', [ 8;]),struct('Name', 'OutputOVLimit','Startbit', [ 0;],'SignalSize', [ 16;],'ByteOrder', 'LittleEndian','ValueType', 'UNSIGNED','Class', 'uint16','Signed', [ 0;],'Factor', [ 0.05;],'Offset', [ 0;],'Min', [ 0;],'Max', [ 3276.75;],'Units', 'V','Comment', '','StartBit', [ 24;]),struct('Name', 'CoolingPlateFaultLim','Startbit', [ 0;],'SignalSize', [ 16;],'ByteOrder', 'LittleEndian','ValueType', 'SIGNED','Class', 'int16','Signed', [ 1;],'Factor', [ 0.1;],'Offset', [ 0;],'Min', [ -3276.8;],'Max', [ 3276.7;],'Units', 'degC','Comment', '','StartBit', [ 8;]),struct('Name', 'CoolingPlateWarningLim','Startbit', [ 0;],'SignalSize', [ 16;],'ByteOrder', 'LittleEndian','ValueType', 'SIGNED','Class', 'int16','Signed', [ 1;],'Factor', [ 0.1;],'Offset', [ 0;],'Min', [ -3276.8;],'Max', [ 3276.7;],'Units', 'degC','Comment', '','StartBit', [ 24;])}}
      settings: SourceProductName=Raptor
  wires:
  Data/1 -> Bus Selector2/1
  CANTxField/1 -> raptor_can_txmsg/1  "OutputCurrentSetpt"
  CANTxField1/1 -> raptor_can_txmsg/2  "OutputVoltageSetpt"
  raptor_adjustment1/1 -> raptor_can_txmsg1/2  "OutputUVLimit"
  raptor_adjustment/1 -> raptor_can_txmsg1/1  "OutputOVLimit"
  raptor_adjustment2/1 -> raptor_can_txmsg2/1  "CoolingPlateFaultLim"
  raptor_adjustment3/1 -> raptor_can_txmsg2/2  "CoolingPlateWarningLim"
  CANTxField2/1 -> raptor_can_txmsg/3  "RemoteShutdown"
  Bus Selector2/1 -> CANTxField/1  "<DCDCOutptCurLim [A]>"
  Bus Selector2/2 -> CANTxField1/1  "<DCDCOutptVoltSetpt [V]>"
  Bus Selector2/3 -> CANTxField2/1  "<DCDCEnblReq [Bool]>"

== system VCMGCM1962020b_v2/Fgnd/Actuators/CAN/DC//DC Converter1/DCDCDCDC_Cmmd_0_16V/MsgTx ==
  Data : Inport
  Enable : EnablePort
  Bus Selector2 : BusSelector  OutputSignals=Control.DCDC.DCDCEnblReq [Bool],Control.DCDC.DCDCOutptCurLim [A],Control.DCDC.DCDCOutptVoltSetpt [V]
  CANTxField : Blocks_lib/CANTxField  custom=on  custom_nam=[nam '---']  custom_units='---'
  CANTxField1 : Blocks_lib/CANTxField  custom=on  custom_nam=[nam '---']  custom_units='---'
  CANTxField2 : Blocks_lib/CANTxField  custom=on  custom_nam=[nam '---']  custom_units='---'
  Header : Blocks_lib/Header  width=Landscape  addtext=''
  raptor_can_txmsg : Raptor_lib/CAN/raptor_can_txmsg  canDefinition=struct('dbcFile', 'Dilong DCDC Converter_dbc file_v2.dbc','message', 'DCDC_Cmmd_0_16V','comment', '','signals', {{'DCDC_Power_cmmd_0_16V','DCDC_Set_Current_0_16V','DCDC_Set_Voltage_0_16V'}},'enabled', [ 1 1 1;],'scaled', [ 1 1 1;],'canBus', 'bus','messageID', [ 402716133;],'idMask', [ 536870911;],'payloadMask', [],'payloadValue', [],'period', [ 100;],'mailbox', '''''','queueSize', [ 1;],'label', [ 1;],'ver', [ 2;],'showID', [ 0;],'showRaw', [ 0;],'fill', [ 0;],'editID', [ 0;],'signalOrder', [ 1;],'signalAscDes', [ 1;])  canBus=bus  queueSize=1  payloadMask=[]  payloadValue=[]  period=100  showID=0  label=1  idMask=hex2dec('1FFFFFFF')  fill=0  id=402716133  showRaw=0  signalOrder=1  signalInfo={{struct('Name', 'DCDC_Power_cmmd_0_16V','Startbit', [ 0;],'SignalSize', [ 1;],'ByteOrder', 'LittleEndian','ValueType', 'UNSIGNED','Class', 'uint8','Signed', [ 0;],'Factor', [ 1;],'Offset', [ 0;],'Min', [ 0;],'Max', [ 1;],'Units', 'enum','Comment', '','StartBit', [ 8;]),struct('Name', 'DCDC_Set_Voltage_0_16V','Startbit', [ 0;],'SignalSize', [ 16;],'ByteOrder', 'LittleEndian','ValueType', 'UNSIGNED','Class', 'uint16','Signed', [ 0;],'Factor', [ 0.1;],'Offset', [ 0;],'Min', [ 0;],'Max', [ 150;],'Units', 'V','Comment', '','StartBit', [ 16;]),struct('Name', 'DCDC_Set_Current_0_16V','Startbit', [ 0;],'SignalSize', [ 16;],'ByteOrder', 'LittleEndian','ValueType', 'UNSIGNED','Class', 'uint16','Signed', [ 0;],'Factor', [ 0.1;],'Offset', [ 0;],'Min', [ 0;],'Max', [ 1500;],'Units', 'A','Comment', '','StartBit', [ 32;])}}
      settings: SourceProductName=Raptor
  wires:
  Data/1 -> Bus Selector2/1
  CANTxField/1 -> raptor_can_txmsg/1  "DCDC_Power_cmmd_0_16V"
  CANTxField1/1 -> raptor_can_txmsg/2  "DCDC_Set_Current_0_16V"
  CANTxField2/1 -> raptor_can_txmsg/3  "DCDC_Set_Voltage_0_16V"
  Bus Selector2/1 -> CANTxField/1  "<DCDCEnblReq [Bool]>"
  Bus Selector2/2 -> CANTxField1/1  "<DCDCOutptCurLim [A]>"
  Bus Selector2/3 -> CANTxField2/1  "<DCDCOutptVoltSetpt [V]>"
